simulink model "angulo_carga"  (R2023b)
settings: Solver=FixedStepAuto  StartTime=0.0  StopTime=10.0  FixedStep=0.001  RelTol=1e-3
undefined symbols (not defined in the file): Y_t0
settings Model: Creator=Ferran  LastModifiedBy=Ferran
settings DebuggingCC: AlgebraicLoopMsg=none  ArtificialAlgebraicLoopMsg=none
settings ModelReferenceCC: ModelReferenceMinAlgLoopOccurrences=on

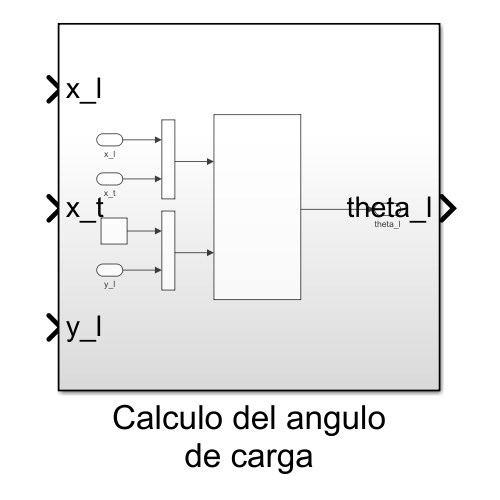
[thumbnail: Simulink's stored preview of the top-level diagram]
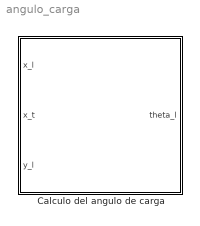
== system angulo_carga ==
  Calculo del angulo de carga : Subsystem

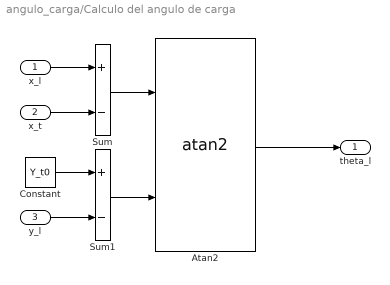
== system angulo_carga/Calculo del angulo de carga ==
  x_l : Inport
  x_t : Inport  Port=2
  y_l : Inport  Port=3
  Atan2 : Trigonometry  Operator=atan2
  Constant : Constant  Value=Y_t0
  Sum : Sum  Inputs=+-
  Sum1 : Sum  Inputs=+-
  theta_l : Outport
  wires:
  x_t/1 -> Sum/2
  Sum1/1 -> Atan2/2
  x_l/1 -> Sum/1
  Sum/1 -> Atan2/1
  Atan2/1 -> theta_l/1
  y_l/1 -> Sum1/2
  Constant/1 -> Sum1/1
